simulink model "Cessna_Altitude_Control_Example"  (R2013a)
settings: Solver=ode45  StartTime=0.0  StopTime=inf  RelTol=1e-3
undefined symbols (not defined in the file): selecting_parameters
libraries: simulink x2, X_Plane_Communication_Library x2
settings Model: Creator=Adriano  LastModifiedBy=Adriano

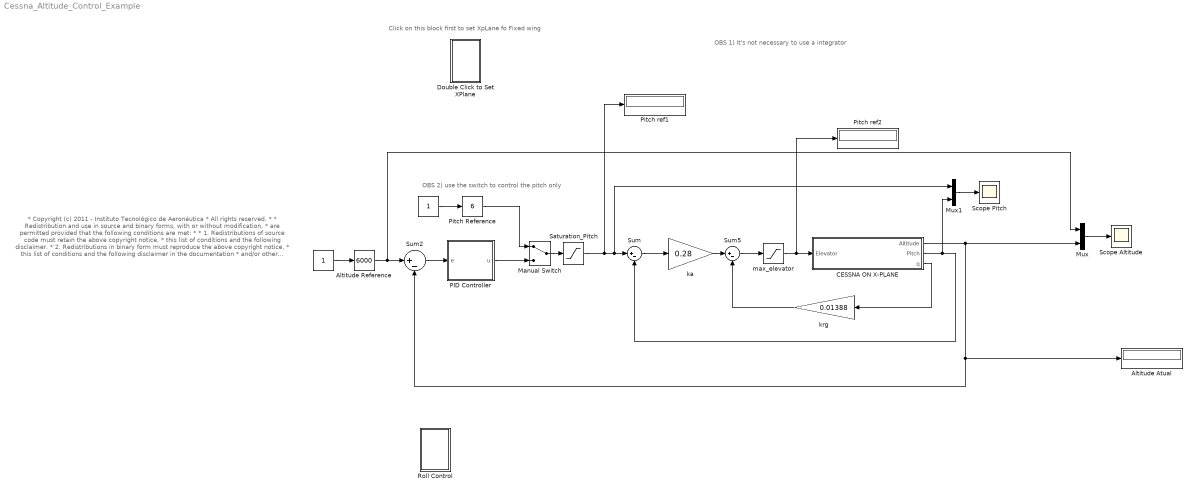
== system Cessna_Altitude_Control_Example ==
  note: Click on this block first to set XpLane fo Fixed wing
  note: * Copyright (c) 2011 -  Instituto Tecnológico de Aeronáutica
      |  * All rights reserved.
      |  *
      |  * Redistribution and use in source and binary forms, with or without modification,
      |  * are permitted provided that the following conditions are met:
      |  *
      |  * 1. Redistributions of source code must retain the above copyright notice,
      |  *    this list of conditions and the following disclaimer.
      |  * 2. Redistributions in binary form must reproduce the above copyright notice,
      |  *    this list of conditions and the following disclaimer in the documentation
      |  *    and/or other materials provided with the distribution.
      |  * 3. The name of the author may not be used to endorse or promote products
      |  *    derived from this software without specific prior written permission.
      |  *
      |  * THIS SOFTWARE IS PROVIDED BY THE AUTHOR ``AS IS'' AND ANY EXPRESS OR IMPLIED
      |  * WARRANTIES, INCLUDING, BUT NOT LIMITED TO, THE IMPLIED WARRANTIES OF
      |  * MERCHANTABILITY AND FITNESS FOR A PARTICULAR PURPOSE ARE DISCLAIMED. IN NO EVENT
      |  * SHALL THE AUTHOR BE LIABLE FOR ANY DIRECT, INDIRECT, INCIDENTAL, SPECIAL,
      |  * EXEMPLARY, OR CONSEQUENTIAL DAMAGES (INCLUDING, BUT NOT LIMITED TO, PROCUREMENT
      |  * OF SUBSTITUTE GOODS OR SERVICES; LOSS OF USE, DATA, OR PROFITS; OR BUSINESS
      |  * INTERRUPTION) HOWEVER CAUSED AND ON ANY THEORY OF LIABILITY, WHETHER IN
      |  * CONTRACT, STRICT LIABILITY, OR TORT (INCLUDING NEGLIGENCE OR OTHERWISE) ARISING
      |  * IN ANY WAY OUT OF THE USE OF THIS SOFTWARE, EVEN IF ADVISED OF THE POSSIBILITY
      |  * OF SUCH DAMAGE.
      |  *
      |  * This file is part of the Pegasus AutoPilot Project
      |  *
      |  * Author: Adriano Bittar <adrianobittar@gmail.com>
      |  *
      |
      |     Pegasus AutoPilot is free software: you can redistribute it and/or modify
      |     it under the terms of the GNU General Public License as published by
      |     the Free Software Foundation, either version 3 of the License, or
      |     any later version.
      |
      |     This program is distributed in the hope that it will be useful,
      |     but WITHOUT ANY WARRANTY; without even the implied warranty of
      |     MERCHANTABILITY or FITNESS FOR A PARTICULAR PURPOSE.  See the
      |     GNU General Public License for more details.
      |
      |     You should have received a copy of the GNU General Public License
      |     along with this program.  If not, see <http://www.gnu.org/licenses/>.
  note: OBS 2) use the switch to control the pitch only
  note: OBS 1) It's not necessary to use a integrator
  " " : Constant
  "    " : Constant
  Altitude Atual : Display
  "Altitude Reference " : simulink/Math Operations/Slider Gain  low=5000  gain=6000  high=10000
  CESSNA ON X-PLANE : Subsystem
  Double Click to Set XPlane : Subsystem  LoadFcn=selecting_parameters()
      settings: OpenFcn=selecting_parameters()
  Manual Switch : ManualSwitch
  Mux : Mux  Inputs=2
  Mux1 : Mux  Inputs=2
  PID Controller : Subsystem
  "Pitch Reference " : simulink/Math Operations/Slider Gain  low=0  gain=6  high=15
  Pitch ref1 : Display
  Pitch ref2 : Display
  Roll Control : Subsystem
  Saturation_Pitch : Saturate  UpperLimit=20  LowerLimit=-20
  Scope Altitude : Scope
      settings: YMin=800  YMax=825
  Scope Pitch : Scope
      settings: YMin=3.8  YMax=6
  Sum : Sum  Inputs=|+-
  Sum2 : Sum  Inputs=|+-  SaturateOnIntegerOverflow=on
  Sum5 : Sum  Inputs=|+-
  ka : Gain  Gain=0.28  OutDataTypeStr=Inherit: Same as input  ParamDataTypeStr=Inherit: Same as input
  krg : Gain  Gain=0.01388  OutDataTypeStr=Inherit: Same as input  ParamDataTypeStr=Inherit: Same as input
  max_elevator : Saturate
  wires:
  Mux/1 -> Scope Altitude/1
  Sum2/1 -> PID Controller/1(e)
  PID Controller/1(u) -> Manual Switch/2
  "    "/1 -> "Pitch Reference "/1
  " "/1 -> "Altitude Reference "/1
  Manual Switch/1 -> Saturation_Pitch/1
  Saturation_Pitch/1 -> Sum/1, Mux1/1, Pitch ref1/1
  ka/1 -> Sum5/1
  krg/1 -> Sum5/2
  Sum/1 -> ka/1
  Sum5/1 -> max_elevator/1
  max_elevator/1 -> CESSNA ON X-PLANE/1(Elevator), Pitch ref2/1
  CESSNA ON X-PLANE/3(q) -> krg/1
  CESSNA ON X-PLANE/2(Pitch) -> Sum/2, Mux1/2
  Mux1/1 -> Scope Pitch/1
  CESSNA ON X-PLANE/1(Altitude) -> Mux/2, Altitude Atual/1, Sum2/2
  "Altitude Reference "/1 -> Sum2/1, Mux/1
  "Pitch Reference "/1 -> Manual Switch/1

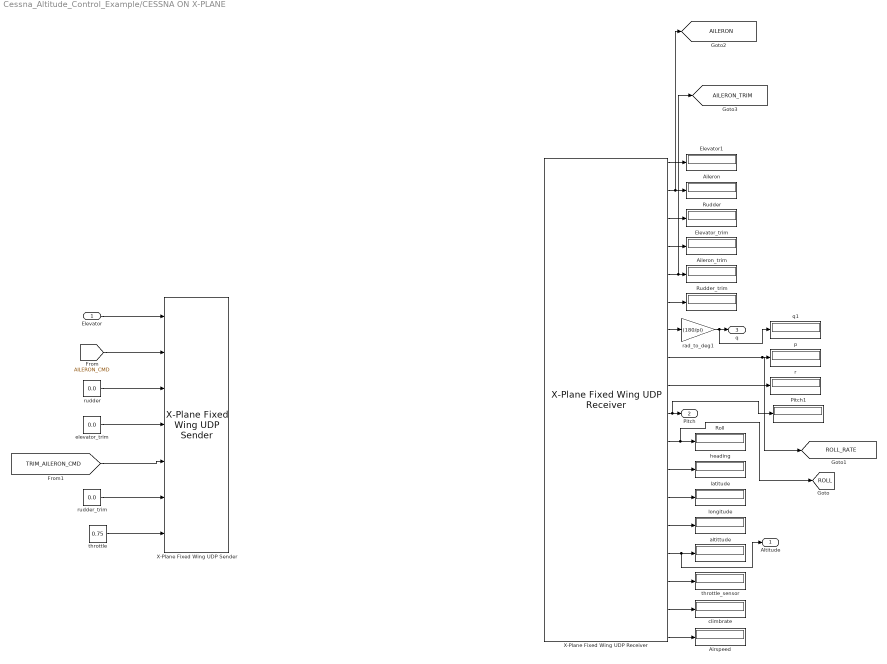
== system Cessna_Altitude_Control_Example/CESSNA ON X-PLANE ==
  Elevator : Inport
  Aileron : Display
  Aileron_trim : Display
  Airspeed : Display
  Elevator1 : Display
  Elevator_trim : Display
  Pitch1 : Display
  Roll : Display
  Rudder : Display
  Rudder_trim : Display
  X-Plane Fixed Wing UDP Receiver : X_Plane_Communication_Library/Fixed Wing/X-Plane Fixed Wing UDP Receiver  ip_adress='127.0.0.1'  port_number=49004
  X-Plane Fixed Wing UDP Sender : X_Plane_Communication_Library/Fixed Wing/X-Plane Fixed Wing UDP Sender  ip_adress='127.0.0.1'  port_number=49000
  altittude : Display
  climbrate : Display
  elevator_trim : Constant  Value=0.0
  heading : Display
  latitude : Display
  longitude : Display
  p : Display
  q1 : Display
  r : Display
  rad_to_deg1 : Gain  Gain=(180/pi)
  rudder : Constant  Value=0.0
  rudder_trim : Constant  Value=0.0
  throttle : Constant  Value=0.75
  throttle_sensor : Display
  Altitude : Outport
  Pitch : Outport  Port=2
  q : Outport  Port=3
  tag scope: AILERON=global, AILERON_TRIM=global, ROLL=global, ROLL_RATE=global
  wires:
  X-Plane Fixed Wing UDP Receiver/7 -> rad_to_deg1/1
  X-Plane Fixed Wing UDP Receiver/10 -> Pitch1/1, Pitch/1
  rad_to_deg1/1 -> q1/1, q/1
  X-Plane Fixed Wing UDP Receiver/1 -> Elevator1/1
  X-Plane Fixed Wing UDP Receiver/2 -> [AILERON], Aileron/1
  X-Plane Fixed Wing UDP Receiver/3 -> Rudder/1
  X-Plane Fixed Wing UDP Receiver/4 -> Elevator_trim/1
  X-Plane Fixed Wing UDP Receiver/5 -> [AILERON_TRIM], Aileron_trim/1
  X-Plane Fixed Wing UDP Receiver/8 -> [ROLL_RATE], p/1
  X-Plane Fixed Wing UDP Receiver/11 -> [ROLL], Roll/1
  X-Plane Fixed Wing UDP Receiver/9 -> r/1
  X-Plane Fixed Wing UDP Receiver/6 -> Rudder_trim/1
  X-Plane Fixed Wing UDP Receiver/12 -> heading/1
  X-Plane Fixed Wing UDP Receiver/13 -> latitude/1
  X-Plane Fixed Wing UDP Receiver/14 -> longitude/1
  X-Plane Fixed Wing UDP Receiver/15 -> Altitude/1, altittude/1
  X-Plane Fixed Wing UDP Receiver/16 -> throttle_sensor/1
  X-Plane Fixed Wing UDP Receiver/17 -> climbrate/1
  X-Plane Fixed Wing UDP Receiver/18 -> Airspeed/1
  Elevator/1 -> X-Plane Fixed Wing UDP Sender/1
  rudder/1 -> X-Plane Fixed Wing UDP Sender/3
  [AILERON_CMD] -> X-Plane Fixed Wing UDP Sender/2
  elevator_trim/1 -> X-Plane Fixed Wing UDP Sender/4
  [TRIM_AILERON_CMD] -> X-Plane Fixed Wing UDP Sender/5
  rudder_trim/1 -> X-Plane Fixed Wing UDP Sender/6
  throttle/1 -> X-Plane Fixed Wing UDP Sender/7

== system Cessna_Altitude_Control_Example/Double Click to Set XPlane ==

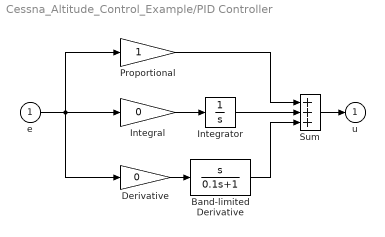
== system Cessna_Altitude_Control_Example/PID Controller ==
  e : Inport
  Band-limited Derivative : TransferFcn  Numerator=[1 0]  Denominator=[0.1 1]
  Derivative : Gain  Gain=0  SaturateOnIntegerOverflow=on  OutDataTypeStr=Inherit: Same as input  ParamDataTypeStr=Inherit: Same as input
  Integral : Gain  Gain=0  SaturateOnIntegerOverflow=on  OutDataTypeStr=Inherit: Same as input  ParamDataTypeStr=Inherit: Same as input
  Integrator : Integrator
  Proportional : Gain  SaturateOnIntegerOverflow=on  OutDataTypeStr=Inherit: Same as input  ParamDataTypeStr=Inherit: Same as input
  Sum : Sum  Inputs=+++  SaturateOnIntegerOverflow=on  InputSameDT=on  OutDataTypeStr=Inherit: Same as first input
  u : Outport  InitialOutput=0
  wires:
  Proportional/1 -> Sum/1
  Integral/1 -> Integrator/1
  Band-limited Derivative/1 -> Sum/3
  e/1 -> Integral/1, Proportional/1, Derivative/1
  Sum/1 -> u/1
  Derivative/1 -> Band-limited Derivative/1
  Integrator/1 -> Sum/2

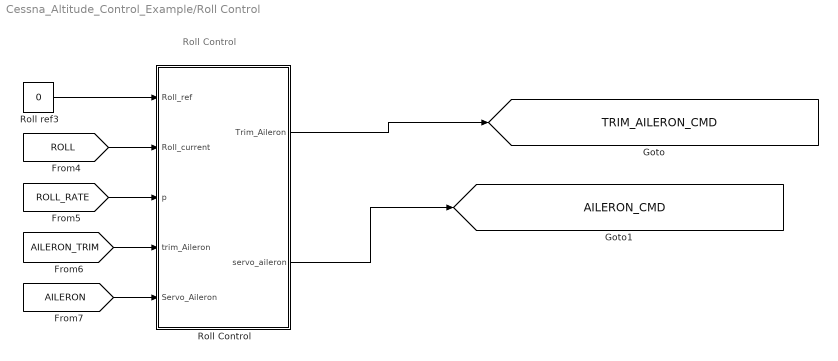
== system Cessna_Altitude_Control_Example/Roll Control ==
  note: Roll Control
  Roll Control : Subsystem
  Roll ref3 : Constant  Value=0
  tag scope: AILERON_CMD=global, TRIM_AILERON_CMD=global
  wires:
  Roll ref3/1 -> Roll Control/1(Roll_ref)
  [AILERON] -> Roll Control/5(Servo_Aileron)
  [AILERON_TRIM] -> Roll Control/4(trim_Aileron)
  [ROLL_RATE] -> Roll Control/3(p)
  [ROLL] -> Roll Control/2(Roll_current)
  Roll Control/1(Trim_Aileron) -> [TRIM_AILERON_CMD]
  Roll Control/2(servo_aileron) -> [AILERON_CMD]

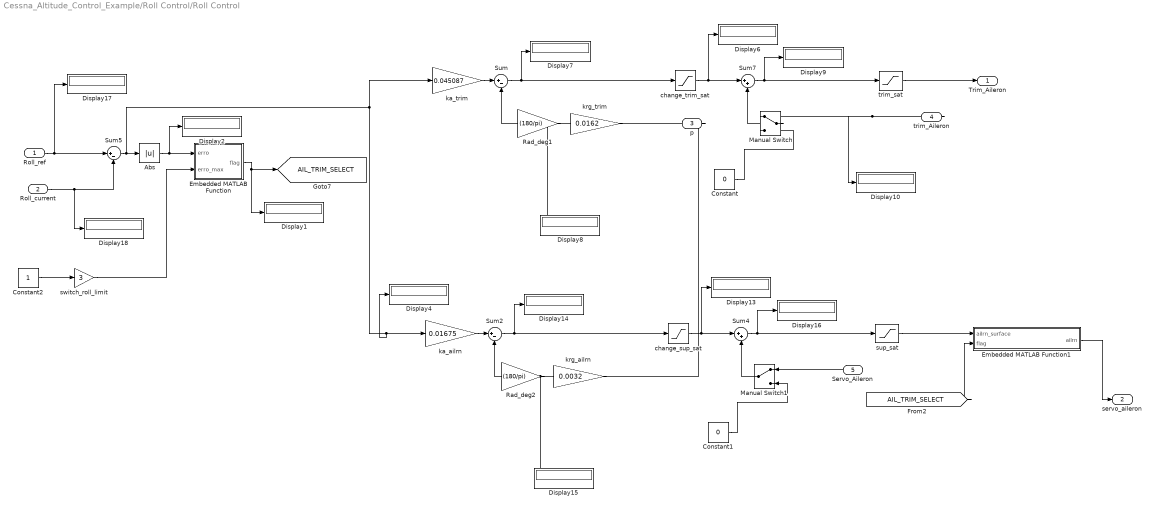
== system Cessna_Altitude_Control_Example/Roll Control/Roll Control ==
  Roll_ref : Inport
  Roll_current : Inport  Port=2
  p : Inport  Port=3
  trim_Aileron : Inport  Port=4
  Servo_Aileron : Inport  Port=5
  Abs : Abs
  Constant : Constant  Value=0
  Constant1 : Constant  Value=0
  Constant2 : Constant
  Display{1..2,4,6..10,13..18} (14 alike) : Display
  Embedded MATLAB Function : MATLAB Function  TreatAsAtomicUnit=on
  Embedded MATLAB Function1 : MATLAB Function  TreatAsAtomicUnit=on
  Manual Switch : ManualSwitch
  Manual Switch1 : ManualSwitch
  Rad_deg1 : Gain  Gain=(180/pi)
  Rad_deg2 : Gain  Gain=(180/pi)
  Sum : Sum  Inputs=|+-
  Sum2 : Sum  Inputs=|+-
  Sum4 : Sum  Inputs=|++
  Sum5 : Sum  Inputs=|+-
  Sum7 : Sum  Inputs=|++
  change_sup_sat : Saturate  UpperLimit=0.1  LowerLimit=-0.1
  change_trim_sat : Saturate  UpperLimit=0.1  LowerLimit=-0.1
  ka_ailrn : Gain  Gain=0.01675  OutDataTypeStr=Inherit: Same as input  ParamDataTypeStr=Inherit: Same as input
  ka_trim : Gain  Gain=0.045087  OutDataTypeStr=Inherit: Same as input  ParamDataTypeStr=Inherit: Same as input
  krg_ailrn : Gain  Gain=0.0032  OutDataTypeStr=Inherit: Same as input  ParamDataTypeStr=Inherit: Same as input
  krg_trim : Gain  Gain=0.0162  OutDataTypeStr=Inherit: Same as input  ParamDataTypeStr=Inherit: Same as input
  sup_sat : Saturate  UpperLimit=0.9  LowerLimit=-0.9  OutMin=-1  OutMax=1  OutDataTypeStr=double  RndMeth=Nearest
  switch_roll_limit : Gain  Gain=3
  trim_sat : Saturate  UpperLimit=1  LowerLimit=-1  OutMin=-1  OutMax=1  OutDataTypeStr=double  RndMeth=Nearest
  Trim_Aileron : Outport
  servo_aileron : Outport  Port=2
  tag scope: AIL_TRIM_SELECT=global
  wires:
  ka_trim/1 -> Sum/1
  Sum/1 -> Display7/1, change_trim_sat/1
  change_trim_sat/1 -> Sum7/1, Display6/1
  Sum7/1 -> Display9/1, trim_sat/1
  krg_trim/1 -> Rad_deg1/1
  p/1 -> krg_trim/1, krg_ailrn/1
  Manual Switch/1 -> Sum7/2
  Constant/1 -> Manual Switch/2
  ka_ailrn/1 -> Sum2/1
  Sum2/1 -> Display14/1, change_sup_sat/1
  change_sup_sat/1 -> Sum4/1, Display13/1
  Sum4/1 -> Display16/1, sup_sat/1
  krg_ailrn/1 -> Rad_deg2/1
  Manual Switch1/1 -> Sum4/2
  Servo_Aileron/1 -> Manual Switch1/1
  Constant1/1 -> Manual Switch1/2
  Roll_ref/1 -> Sum5/1, Display17/1
  Roll_current/1 -> Sum5/2, Display18/1
  Sum5/1 -> Abs/1, ka_trim/1, ka_ailrn/1, Display4/1
  switch_roll_limit/1 -> Embedded MATLAB Function/2(erro_max)
  Constant2/1 -> switch_roll_limit/1
  Abs/1 -> Embedded MATLAB Function/1(erro), Display2/1
  Rad_deg2/1 -> Sum2/2, Display15/1
  Rad_deg1/1 -> Sum/2, Display8/1
  Embedded MATLAB Function/1(flag) -> Display1/1, [AIL_TRIM_SELECT]
  trim_Aileron/1 -> Manual Switch/1, Display10/1
  trim_sat/1 -> Trim_Aileron/1
  sup_sat/1 -> Embedded MATLAB Function1/1(ailrn_surface)
  [AIL_TRIM_SELECT] -> Embedded MATLAB Function1/2(flag)
  Embedded MATLAB Function1/1(ailrn) -> servo_aileron/1

== matlab function Cessna_Altitude_Control_Example/Roll Control/Roll Control/Embedded MATLAB Function1 ==
  data: ailrn_surface input; flag input; ailrn output
function ailrn   = fcn_elev(ailrn_surface,flag)
% This block supports the Embedded MATLAB subset.
% See the help menu for details. 

if(flag == 1)
   
    ailrn = 0;
else
  
   ailrn = ailrn_surface;
end

== matlab function Cessna_Altitude_Control_Example/Roll Control/Roll Control/Embedded MATLAB Function ==
  data: flag output; erro input; erro_max input
function flag = fcn(erro,erro_max)
% This block supports the Embedded MATLAB subset.
% See the help menu for details. 
if(erro<erro_max)
    flag = 1;
else
    flag = 2;
end;
